simulink model "drivetrain_simple_plant"  (R2023b)
settings: Solver=VariableStepAuto  StartTime=0.0  StopTime=10.0  RelTol=1e-3
model workspace (MAT data in the model file):
  B_dt = 0
  J = 1
settings Model: ParameterArgumentNames=B_dt,J  Creator=jaz43  LastModifiedBy=jaz43

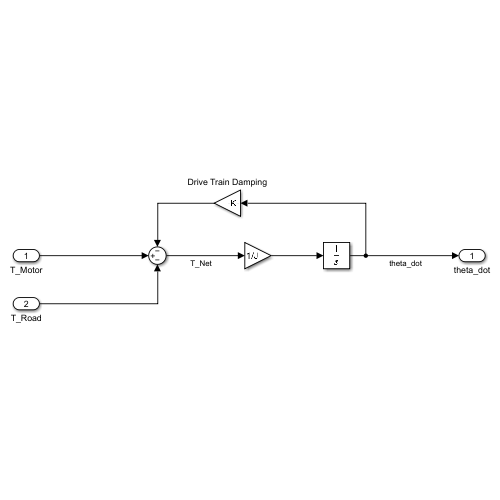
[thumbnail: Simulink's stored preview of the top-level diagram]
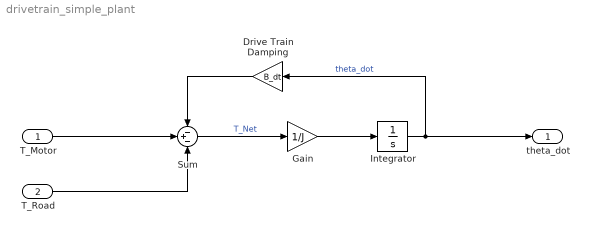
== system drivetrain_simple_plant ==
  T_Motor : Inport
  T_Road : Inport  Port=2
  Drive Train Damping : Gain  Gain=B_dt
  Gain : Gain  Gain=1/J
  Integrator : Integrator
  Sum : Sum  Inputs=-+-
  theta_dot : Outport
  wires:
  Integrator/1 -> theta_dot/1, Drive Train Damping/1  "theta_dot"
  Drive Train Damping/1 -> Sum/1
  T_Motor/1 -> Sum/2
  T_Road/1 -> Sum/3
  Sum/1 -> Gain/1  "T_Net"
  Gain/1 -> Integrator/1
